simulink model "intel_motor_control_rlfreddie"  (Simulink 10.3)
settings: Solver=FixedStepDiscrete  StartTime=0.0  StopTime=0.7  FixedStep=62.5e-6 % 16 kHz  RelTol=1e-3  EnableMultiTasking=on
undefined symbols (not defined in the file or in its folder): DiscIntNeverNeededParam, I_max, Position_PI_Limit
libraries: simulink x9, dspsrcs4 x2, rllib x1
(part 2 of 2)

== system intel_motor_control_rlfreddie/Controller_3phase/Field_Oriented_Control/FOC_SimulinkFloat/FOC_Simulink_float/InverseParkTransform ==
  note: Forward Park Transform: Iq = -IAlpha*Sin(Phi) + IBeta*Cos(Phi)
  note: Forward Park Transform: Id = IAlpha*Cos(Phi) + IBeta*Sin(Phi)
  note: Reverse Park Transform: VAlphaCmd_V = VdCmd_V*Cos(Phi) - VqCmd_V*Sin(Phi)
  note: Reverse Park Transform: VBetaCmd_V = VdCmd_V*Sin(Phi) + VqCmd_V*Cos(Phi)
  VdCmd_V : Inport
  VqCmd_V : Inport  Port=2
  SinPhi_ND : Inport  Port=3
  CosPhi_ND : Inport  Port=4
  CosPhi_ND1 : InportShadow  Port=4
  Product{,1..3} (4 alike) : Product
  SinPhi_ND1 : InportShadow  Port=3
  Sum : Sum  Inputs=|+-
  Sum1 : Sum  Inputs=|++
  VdCmd_V1 : InportShadow
  VqCmd_V1 : InportShadow  Port=2
  VAlphaCmd_V : Outport
  VBetaCmd_V : Outport  Port=2
  wires:
  Sum1/1 -> VBetaCmd_V/1
  Product3/1 -> Sum1/2
  Product2/1 -> Sum1/1
  CosPhi_ND1/1 -> Product3/2
  VqCmd_V1/1 -> Product3/1
  SinPhi_ND1/1 -> Product2/2
  VdCmd_V1/1 -> Product2/1
  Sum/1 -> VAlphaCmd_V/1
  Product1/1 -> Sum/2
  Product/1 -> Sum/1
  SinPhi_ND/1 -> Product1/2
  CosPhi_ND/1 -> Product/2
  VdCmd_V/1 -> Product/1
  VqCmd_V/1 -> Product1/1

== system intel_motor_control_rlfreddie/Controller_3phase/Field_Oriented_Control/FOC_SimulinkFloat/FOC_Simulink_float/ParkTransform ==
  note: Id = IAlpha*Cos(Phi) + IBeta*Sin(Phi)
  note: Iq = -IAlpha*Sin(Phi) + IBeta*Cos(Phi)
  IAlpha_A : Inport
  IBeta_A : Inport  Port=2
  SinPhi_ND : Inport  Port=3
  CosPhi_ND : Inport  Port=4
  CosPhi_ND1 : InportShadow  Port=4
  IAlpha_A1 : InportShadow
  IBeta_A1 : InportShadow  Port=2
  Product{,1..3} (4 alike) : Product
  SinPhi_ND1 : InportShadow  Port=3
  Sum : Sum  Inputs=|++
  Sum1 : Sum  Inputs=|-+
  Id_A : Outport
  Iq_A : Outport  Port=2
  wires:
  IBeta_A/1 -> Product1/1
  IAlpha_A/1 -> Product/1
  CosPhi_ND/1 -> Product/2
  SinPhi_ND/1 -> Product1/2
  Product/1 -> Sum/1
  Product1/1 -> Sum/2
  Sum/1 -> Id_A/1
  IAlpha_A1/1 -> Product2/1
  SinPhi_ND1/1 -> Product2/2
  IBeta_A1/1 -> Product3/1
  CosPhi_ND1/1 -> Product3/2
  Product2/1 -> Sum1/1
  Product3/1 -> Sum1/2
  Sum1/1 -> Iq_A/1

== system intel_motor_control_rlfreddie/Controller_3phase/Field_Oriented_Control/FOC_SimulinkFloat/FOC_Simulink_float/TwoPIControllers ==
  IdCmd_A_f : Inport
  IqCmd_A_f : Inport  Port=2
  IdFb_A_f : Inport  Port=3
  IqFb_A_f : Inport  Port=4
  FbErrorLimit_A_f : Inport  Port=5
  Kp_ND_f : Inport  Port=6
  Ki_NDperUpdate_f : Inport  Port=7
  IntegratorLimit_f : Inport  Port=8
  CmdLimit_f : Inport  Port=9
  DoReset_Bool : Inport  Port=10
  FbErrorLimit1_A_f : InportShadow  Port=5
  IntegratorLimit1 : InportShadow  Port=8
  Ki_NDperUpdate1 : InportShadow  Port=7
  Kp_ND1 : InportShadow  Port=6
  OutputLimit1 : InportShadow  Port=9
  PIController : Subsystem
  PIController1 : Subsystem
  ResetState_Bool1 : InportShadow  Port=10
  VdUnfilt_V : Outport
  VqUnfilt_V : Outport  Port=2
  wires:
  IdCmd_A_f/1 -> PIController/1(Cmd_f)
  PIController/1(NextCmd_f) -> VdUnfilt_V/1
  IdFb_A_f/1 -> PIController/2(Fb_f)
  PIController1/1(NextCmd_f) -> VqUnfilt_V/1
  ResetState_Bool1/1 -> PIController1/8(DoReset_Bool)
  OutputLimit1/1 -> PIController1/7(CmdLimit_f)
  IntegratorLimit1/1 -> PIController1/6(IntegratorLimit_f)
  Ki_NDperUpdate1/1 -> PIController1/5(Ki_NDperUpdate_f)
  Kp_ND1/1 -> PIController1/4(Kp_ND_f)
  FbErrorLimit1_A_f/1 -> PIController1/3(FbErrorLimit_f)
  IqFb_A_f/1 -> PIController1/2(Fb_f)
  IqCmd_A_f/1 -> PIController1/1(Cmd_f)
  DoReset_Bool/1 -> PIController/8(DoReset_Bool)
  CmdLimit_f/1 -> PIController/7(CmdLimit_f)
  IntegratorLimit_f/1 -> PIController/6(IntegratorLimit_f)
  Ki_NDperUpdate_f/1 -> PIController/5(Ki_NDperUpdate_f)
  Kp_ND_f/1 -> PIController/4(Kp_ND_f)
  FbErrorLimit_A_f/1 -> PIController/3(FbErrorLimit_f)

== system intel_motor_control_rlfreddie/Controller_equiv_DC_motor1/PI_Ctrl_float_speed/Reinforcement Learning1/Observations/limit_abs_value_of_integrator ==
  input : Inport
  abs_max : Inport  Port=2
  CmpLT : RelationalOperator  Operator=<  OutDataTypeStr=boolean  RndMeth=Nearest
  CmpLT1 : RelationalOperator  OutDataTypeStr=boolean  RndMeth=Nearest
  Switch : Switch  Criteria=u2 ~= 0  Threshold=Position_PI_Limit  ZeroCross=off
  Switch1 : Switch  Criteria=u2 ~= 0  Threshold=I_max  ZeroCross=off
  Unary Minus : UnaryMinus
  output : Outport
  wires:
  CmpLT1/1 -> Switch/2
  abs_max/1 -> Switch/1, CmpLT1/2, Unary Minus/1
  input/1 -> CmpLT1/1, Switch/3, CmpLT/1
  CmpLT/1 -> Switch1/2
  Switch/1 -> Switch1/3
  Switch1/1 -> output/1
  Unary Minus/1 -> Switch1/1, CmpLT/2

== system intel_motor_control_rlfreddie/Controller_equiv_DC_motor1/PI_Ctrl_float_speed/Reinforcement Learning1/Reward/limit_abs_value_of_integrator ==
  input : Inport
  abs_max : Inport  Port=2
  CmpLT : RelationalOperator  Operator=<  OutDataTypeStr=boolean  RndMeth=Nearest
  CmpLT1 : RelationalOperator  OutDataTypeStr=boolean  RndMeth=Nearest
  Switch : Switch  Criteria=u2 ~= 0  Threshold=Position_PI_Limit  ZeroCross=off
  Switch1 : Switch  Criteria=u2 ~= 0  Threshold=I_max  ZeroCross=off
  Unary Minus : UnaryMinus
  output : Outport
  wires:
  CmpLT1/1 -> Switch/2
  abs_max/1 -> Switch/1, CmpLT1/2, Unary Minus/1
  input/1 -> CmpLT1/1, Switch/3, CmpLT/1
  CmpLT/1 -> Switch1/2
  Switch/1 -> Switch1/3
  Switch1/1 -> output/1
  Unary Minus/1 -> Switch1/1, CmpLT/2

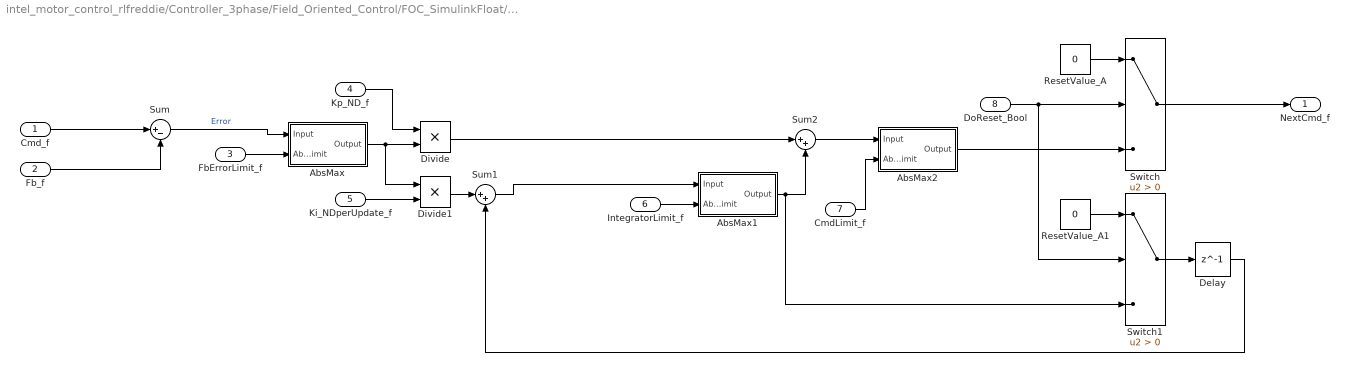
== system intel_motor_control_rlfreddie/Controller_3phase/Field_Oriented_Control/FOC_SimulinkFloat/FOC_Simulink_float/TwoPIControllers/PIController ==
  Cmd_f : Inport
  Fb_f : Inport  Port=2
  FbErrorLimit_f : Inport  Port=3
  Kp_ND_f : Inport  Port=4
  Ki_NDperUpdate_f : Inport  Port=5
  IntegratorLimit_f : Inport  Port=6
  CmdLimit_f : Inport  Port=7
  DoReset_Bool : Inport  Port=8
  AbsMax : Subsystem
  AbsMax1 : Subsystem
  AbsMax2 : Subsystem
  Delay : Delay  DelayLength=1  InitialCondition=0
  Divide : Product  Inputs=**
  Divide1 : Product  Inputs=**
  ResetValue_A : Constant  Value=0
  ResetValue_A1 : Constant  Value=0
  Sum : Sum  Inputs=|+-
  Sum1 : Sum  Inputs=|++
  Sum2 : Sum  Inputs=|++
  Switch : Switch  Criteria=u2 > Threshold
  Switch1 : Switch  Criteria=u2 > Threshold
  NextCmd_f : Outport
  wires:
  Fb_f/1 -> Sum/2
  Cmd_f/1 -> Sum/1
  Ki_NDperUpdate_f/1 -> Divide1/2
  Sum/1 -> AbsMax/1(Input)  "Error"
  Divide1/1 -> Sum1/1
  Kp_ND_f/1 -> Divide/1
  FbErrorLimit_f/1 -> AbsMax/2(AbsLimit)
  Sum1/1 -> AbsMax1/1(Input)
  Divide/1 -> Sum2/1
  AbsMax/1(Output) -> Divide1/1, Divide/2
  Delay/1 -> Sum1/2
  ResetValue_A1/1 -> Switch1/1
  CmdLimit_f/1 -> AbsMax2/2(AbsLimit)
  Sum2/1 -> AbsMax2/1(Input)
  AbsMax1/1(Output) -> Switch1/3, Sum2/2
  Switch/1 -> NextCmd_f/1
  ResetValue_A/1 -> Switch/1
  DoReset_Bool/1 -> Switch1/2, Switch/2
  AbsMax2/1(Output) -> Switch/3
  Switch1/1 -> Delay/1
  IntegratorLimit_f/1 -> AbsMax1/2(AbsLimit)

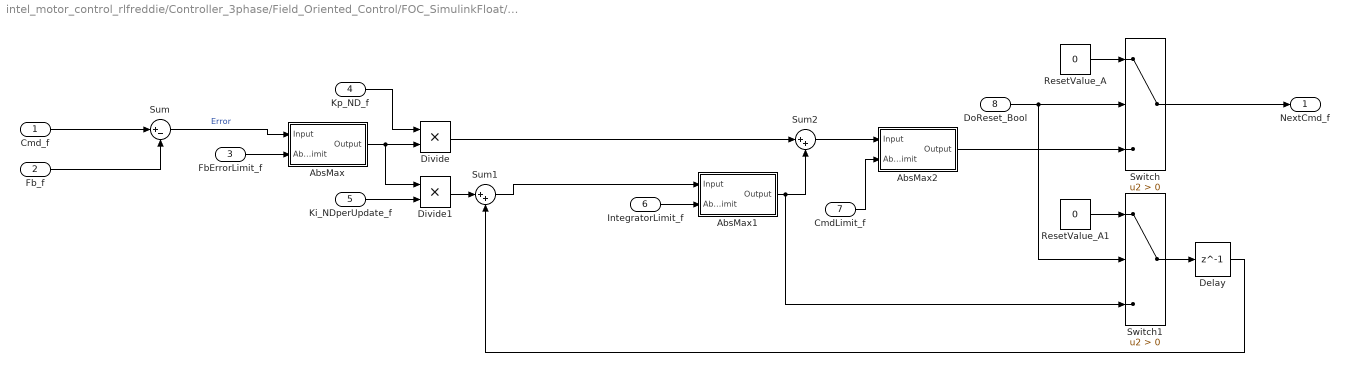
== system intel_motor_control_rlfreddie/Controller_3phase/Field_Oriented_Control/FOC_SimulinkFloat/FOC_Simulink_float/TwoPIControllers/PIController1 ==
  Cmd_f : Inport
  Fb_f : Inport  Port=2
  FbErrorLimit_f : Inport  Port=3
  Kp_ND_f : Inport  Port=4
  Ki_NDperUpdate_f : Inport  Port=5
  IntegratorLimit_f : Inport  Port=6
  CmdLimit_f : Inport  Port=7
  DoReset_Bool : Inport  Port=8
  AbsMax : Subsystem
  AbsMax1 : Subsystem
  AbsMax2 : Subsystem
  Delay : Delay  DelayLength=1  InitialCondition=0
  Divide : Product  Inputs=**
  Divide1 : Product  Inputs=**
  ResetValue_A : Constant  Value=0
  ResetValue_A1 : Constant  Value=0
  Sum : Sum  Inputs=|+-
  Sum1 : Sum  Inputs=|++
  Sum2 : Sum  Inputs=|++
  Switch : Switch  Criteria=u2 > Threshold
  Switch1 : Switch  Criteria=u2 > Threshold
  NextCmd_f : Outport
  wires:
  IntegratorLimit_f/1 -> AbsMax1/2(AbsLimit)
  Switch1/1 -> Delay/1
  AbsMax2/1(Output) -> Switch/3
  DoReset_Bool/1 -> Switch/2, Switch1/2
  ResetValue_A/1 -> Switch/1
  Switch/1 -> NextCmd_f/1
  AbsMax1/1(Output) -> Sum2/2, Switch1/3
  Sum2/1 -> AbsMax2/1(Input)
  CmdLimit_f/1 -> AbsMax2/2(AbsLimit)
  ResetValue_A1/1 -> Switch1/1
  Delay/1 -> Sum1/2
  AbsMax/1(Output) -> Divide/2, Divide1/1
  Divide/1 -> Sum2/1
  Sum1/1 -> AbsMax1/1(Input)
  FbErrorLimit_f/1 -> AbsMax/2(AbsLimit)
  Kp_ND_f/1 -> Divide/1
  Divide1/1 -> Sum1/1
  Sum/1 -> AbsMax/1(Input)  "Error"
  Ki_NDperUpdate_f/1 -> Divide1/2
  Cmd_f/1 -> Sum/1
  Fb_f/1 -> Sum/2

== system intel_motor_control_rlfreddie/Controller_3phase/Field_Oriented_Control/FOC_SimulinkFloat/FOC_Simulink_float/TwoPIControllers/PIController/AbsMax ==
  Input : Inport
  AbsLimit : Inport  Port=2
  Abs : Abs
  Divide : Product  Inputs=**
  Min : MinMax  Inputs=2
  Sign : Signum
  Output : Outport
  wires:
  AbsLimit/1 -> Min/2
  Abs/1 -> Min/1
  Divide/1 -> Output/1
  Min/1 -> Divide/1
  Sign/1 -> Divide/2
  Input/1 -> Sign/1, Abs/1

== system intel_motor_control_rlfreddie/Controller_3phase/Field_Oriented_Control/FOC_SimulinkFloat/FOC_Simulink_float/TwoPIControllers/PIController/AbsMax1 ==
  Input : Inport
  AbsLimit : Inport  Port=2
  Abs : Abs
  Divide : Product  Inputs=**
  Min : MinMax  Inputs=2
  Sign : Signum
  Output : Outport
  wires:
  Input/1 -> Abs/1, Sign/1
  Sign/1 -> Divide/2
  Min/1 -> Divide/1
  Divide/1 -> Output/1
  Abs/1 -> Min/1
  AbsLimit/1 -> Min/2

== system intel_motor_control_rlfreddie/Controller_3phase/Field_Oriented_Control/FOC_SimulinkFloat/FOC_Simulink_float/TwoPIControllers/PIController/AbsMax2 ==
  Input : Inport
  AbsLimit : Inport  Port=2
  Abs : Abs
  Divide : Product  Inputs=**
  Min : MinMax  Inputs=2
  Sign : Signum
  Output : Outport
  wires:
  AbsLimit/1 -> Min/2
  Abs/1 -> Min/1
  Divide/1 -> Output/1
  Min/1 -> Divide/1
  Sign/1 -> Divide/2
  Input/1 -> Sign/1, Abs/1

== system intel_motor_control_rlfreddie/Controller_3phase/Field_Oriented_Control/FOC_SimulinkFloat/FOC_Simulink_float/TwoPIControllers/PIController1/AbsMax ==
  Input : Inport
  AbsLimit : Inport  Port=2
  Abs : Abs
  Divide : Product  Inputs=**
  Min : MinMax  Inputs=2
  Sign : Signum
  Output : Outport
  wires:
  Input/1 -> Abs/1, Sign/1
  Sign/1 -> Divide/2
  Min/1 -> Divide/1
  Divide/1 -> Output/1
  Abs/1 -> Min/1
  AbsLimit/1 -> Min/2

== system intel_motor_control_rlfreddie/Controller_3phase/Field_Oriented_Control/FOC_SimulinkFloat/FOC_Simulink_float/TwoPIControllers/PIController1/AbsMax1 ==
  Input : Inport
  AbsLimit : Inport  Port=2
  Abs : Abs
  Divide : Product  Inputs=**
  Min : MinMax  Inputs=2
  Sign : Signum
  Output : Outport
  wires:
  AbsLimit/1 -> Min/2
  Abs/1 -> Min/1
  Divide/1 -> Output/1
  Min/1 -> Divide/1
  Sign/1 -> Divide/2
  Input/1 -> Sign/1, Abs/1

== system intel_motor_control_rlfreddie/Controller_3phase/Field_Oriented_Control/FOC_SimulinkFloat/FOC_Simulink_float/TwoPIControllers/PIController1/AbsMax2 ==
  Input : Inport
  AbsLimit : Inport  Port=2
  Abs : Abs
  Divide : Product  Inputs=**
  Min : MinMax  Inputs=2
  Sign : Signum
  Output : Outport
  wires:
  Input/1 -> Abs/1, Sign/1
  Sign/1 -> Divide/2
  Min/1 -> Divide/1
  Divide/1 -> Output/1
  Abs/1 -> Min/1
  AbsLimit/1 -> Min/2
